simulink model "fdi"  (R2026a)
settings: Solver=VariableStepAuto

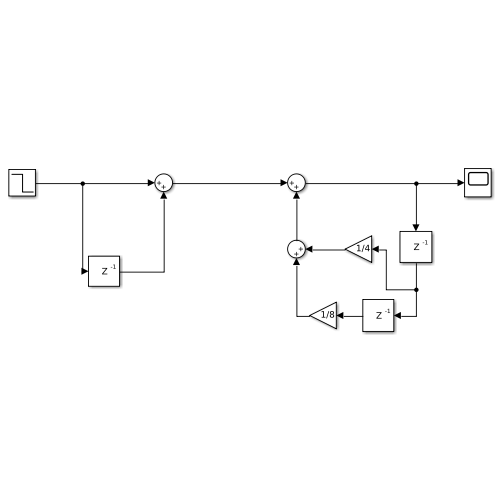
[thumbnail: Simulink's stored preview of the top-level diagram]
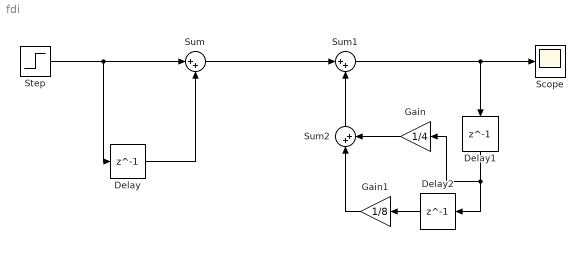
== system fdi ==
  Delay : Delay  DelayLength=1
  Delay1 : Delay  DelayLength=1
  Delay2 : Delay  DelayLength=1
  Gain : Gain  Gain=1/4
  Gain1 : Gain  Gain=1/8
  Scope : Scope
  Step : Step  Time=0  FinalValue=-2  SampleTime=1
  Sum : Sum  Inputs=|++
  Sum1 : Sum  Inputs=|++
  Sum2 : Sum  Inputs=|++
  wires:
  Delay/1 -> Sum/2
  Sum/1 -> Sum1/1
  Sum1/1 -> Scope/1, Delay1/1
  Delay1/1 -> Gain/1, Delay2/1
  Delay2/1 -> Gain1/1
  Gain/1 -> Sum2/2
  Gain1/1 -> Sum2/1
  Sum2/1 -> Sum1/2
  Step/1 -> Delay/1, Sum/1
